simulink model "F11_implementation"  (R2017a)
settings: Solver=VariableStepAuto  StartTime=0.0  StopTime=100  FixedStep=.025  RelTol=1e-3
undefined symbols (not defined in the file or in its folder): F_animation, P
libraries: simulink x1
settings Model: Creator=Mat Haskell  LastModifiedBy=Mat Haskell

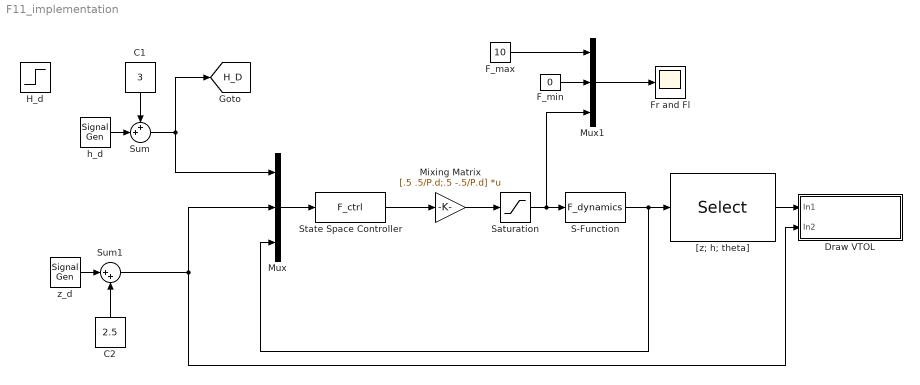
== system F11_implementation ==
  C1 : Constant  Value=3
  C2 : Constant  Value=2.5
  Draw VTOL : Subsystem
  F_max : Constant  Value=10
  F_min : Constant  Value=0
  Fr and Fl : Scope
  H_d : Step  Time=0  After=0  SampleTime=0
  Mixing Matrix : Gain  Gain=[.5 .5/P.d;.5 -.5/P.d]  Multiplication=Matrix(K*u)
  Mux : Mux  Inputs=3
  Mux1 : Mux  Inputs=3
  S-Function : S-Function  FunctionName=F_dynamics  Parameters=P  SFunctionDeploymentMode=off  EnableBusSupport=off
  Saturation : Saturate  UpperLimit=10  LowerLimit=0
  State Space Controller : MATLABFcn  MATLABFcn=F_ctrl
  Sum : Sum  Inputs=++|
  Sum1 : Sum  Inputs=|++
  "[z; h; theta]" : Selector  InputPortWidth=6  IndexOptions=Index vector (dialog)  Indices=[1 2 3]  OutputSizes=1
  h_d : SignalGenerator  WaveForm=square  Amplitude=2  Frequency=.05
  z_d : SignalGenerator  WaveForm=square  Amplitude=2.5  Frequency=.04
  tag scope: H_D=global
  wires:
  C1/1 -> Sum/1
  Sum/1 -> Mux/1, [H_D]
  z_d/1 -> Sum1/1
  C2/1 -> Sum1/2
  Sum1/1 -> Mux/2, Draw VTOL/2(In2)
  State Space Controller/1 -> Mixing Matrix/1
  S-Function/1 -> Mux/3, "[z; h; theta]"/1
  Mixing Matrix/1 -> Saturation/1
  Mux1/1 -> Fr and Fl/1
  F_min/1 -> Mux1/2
  F_max/1 -> Mux1/1
  Saturation/1 -> Mux1/3, S-Function/1
  h_d/1 -> Sum/2
  Mux/1 -> State Space Controller/1
  "[z; h; theta]"/1 -> Draw VTOL/1(In1)

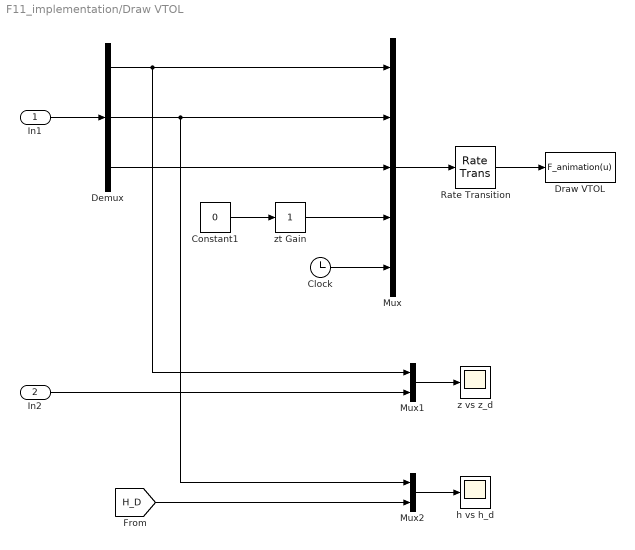
== system F11_implementation/Draw VTOL ==
  In1 : Inport
  In2 : Inport  Port=2
  Clock : Clock
  Constant1 : Constant  Value=0
  Demux : Demux  Outputs=3
  Draw VTOL : MATLABFcn  InitFcn=|  MATLABFcn=F_animation(u)  OutputDimensions=0
      | clear;clc
      | F_param
  Mux : Mux  Inputs=5
  Mux1 : Mux  Inputs=2
  Mux2 : Mux  Inputs=2
  Rate Transition : RateTransition  OutPortSampleTime=P.t_plot
  h vs h_d : Scope
  z vs z_d : Scope
  zt Gain : simulink/Math Operations/Slider Gain  gain=1  low=0  high=5
  wires:
  In1/1 -> Demux/1
  Demux/1 -> Mux1/1, Mux/1
  Demux/2 -> Mux2/1, Mux/2
  Demux/3 -> Mux/3
  Rate Transition/1 -> Draw VTOL/1
  Mux/1 -> Rate Transition/1
  zt Gain/1 -> Mux/4
  Constant1/1 -> zt Gain/1
  Clock/1 -> Mux/5
  In2/1 -> Mux1/2
  Mux1/1 -> z vs z_d/1
  Mux2/1 -> h vs h_d/1
  [H_D] -> Mux2/2
